simulink model "sem7_model"  (R2018b)
settings: Solver=VariableStepAuto  StartTime=0.0  StopTime=inf  RelTol=1e-3
libraries: xpcutilitieslib x2, xpcrtudplib x2, sldrtlib x1, slrtlib x1
settings Model: Creator=117-11  LastModifiedBy=117-11

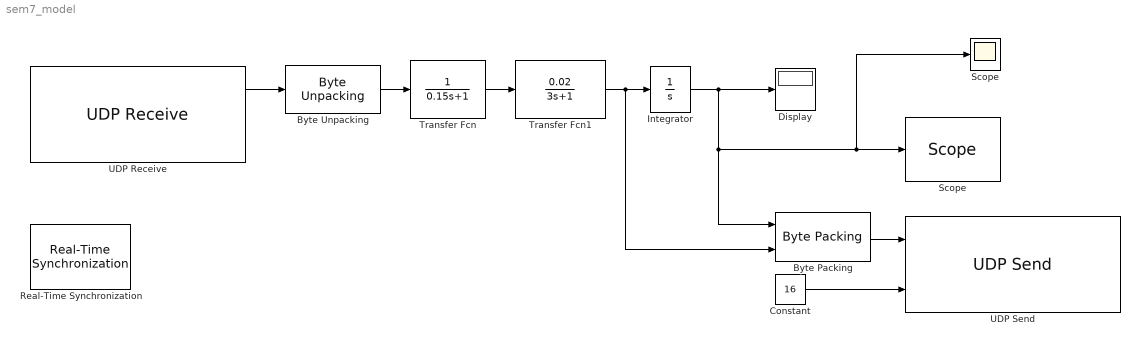
== system sem7_model ==
  "Byte Packing " : xpcutilitieslib/Byte Packing   MaskPackedDataType=uint8  MaskUnpackedDataTypes={'double', 'double'}  MaskAlignment=1
  "Byte Unpacking " : xpcutilitieslib/Byte Unpacking   MaskUnpackedDataTypes={'double'}  MaskUnpackedDataSizes={[1]}  MaskAlignment=1
      settings: SourceProductName=Simulink Real-Time  SourceProductBaseCode=XP
  Constant : Constant  Value=16
  Display : Display
  Integrator : Integrator
  Real-Time Synchronization : sldrtlib/Real-Time Synchronization  SampleTime=0.00001  MaxMissedTicks=10  ShowMissedTicks=off  YieldWhenWaiting=off
  Scope : Scope
  "Scope " : slrtlib/Displays and Logging/Scope   scopeno=1  scopetype=Target  autostart=on  viewmode=Graphical redraw  formatstr='%15.6f'  grid=on  ylimits=[0,0]  nosamples=250  noprepostsamples=0  interleave=1  triggermode=FreeRun  triggersignal=1  trigsignalfromport=off  triggerlevel=0.0  triggerslope=Either  triggerscope=1  triggersample=0  filename=data.dat  mode=Lazy  writesize=512  autorestart=off  dynamicfilemode=off  maxwritefilesize=512*1024^2
  Transfer Fcn : TransferFcn  Denominator=[0.15 1]
  Transfer Fcn1 : TransferFcn  Numerator=[0.02]  Denominator=[3 1]
  UDP Receive : xpcrtudplib/UDP Receive  ipAddressVal=Use host-target connection  localPort=13042  rcvWidth=8  rcvFmAny=on  fmAddress=0.0.0.0  rcvMulticast=off  multicastAddress={}  maxUDPQueue=8  sampleTime=-1
      settings: SourceProductName=Simulink Real-Time
  UDP Send : xpcrtudplib/UDP Send  ipAddressVal=Use host-target connection  localPort=13043  toAddress=127.0.0.1  toPort=13044  sampleTime=0.1
      settings: SourceProductName=Simulink Real-Time  SourceProductBaseCode=XP
  wires:
  "Byte Unpacking "/1 -> Transfer Fcn/1
  UDP Receive/1 -> "Byte Unpacking "/1
  Transfer Fcn/1 -> Transfer Fcn1/1
  Transfer Fcn1/1 -> "Byte Packing "/2, Integrator/1
  Integrator/1 -> "Byte Packing "/1, Scope/1, "Scope "/1, Display/1
  Constant/1 -> UDP Send/2
  "Byte Packing "/1 -> UDP Send/1
